simulink model "power_kundur_statcom01"  (R2021a)
settings: Solver=ode23tb  StartTime=0.0  StopTime=10  MaxStep=1/60  RelTol=1e-4  EnableMultiTasking=on
values from neighbouring files (symbols this model uses):
  j = 1    [OABC_PSO_TUNED_NOFault.mat]    (also in OABC_PSO_TUNED_ThreePHASEFault.mat; Traditional_ABC_PSO2.m = randi([1 noFood], 1))
  kk = [0 0.302628193662]    [OABC_PSO_TUNED_NOFault.mat]    (also in OABC_PSO_TUNED_ThreePHASEFault.mat = [6.69502367045 1584.585174])
undefined symbols (not defined in the file or in its folder): Ac, Bc, Cc, D1, Dc, Delta, Fnom, gcbh, K_Vdq2m_SH, Kf_I_SH, Ki_I_SH, Ki_Vac_SH, Ki_Vdc_SH, Kp_I_SH, Kp_Vac_SH, Kp_Vdc_SH, L_RL_SH, MagIinit_SH, PhaIinit_SH, R_RL_SH, sps_rtmsupport, VdcRef_SH, Vnom_SH, xfo_ratio_SH
libraries: spsGenericPowerSystemStabilizerLib x8, spsLoadFlowBusLib x6, spsThreePhaseParallelRLCLoadLib x4, spsThreePhasePISectionLineLib x4, spsSynchronousMachinepuStandardLib x4, spsExcitationSystemLib x4, spsMultiBandPowerSystemStabilizerLib x4, spsSteamTurbineandGovernorLib x4, spsThreePhaseTransformerTwoWindingsLib x4, spsThreePhaseVIMeasurementLib x3, spsThreePhaseBreakerLib x2, spsControlledCurrentSourceLib x2
(part 2 of 3)

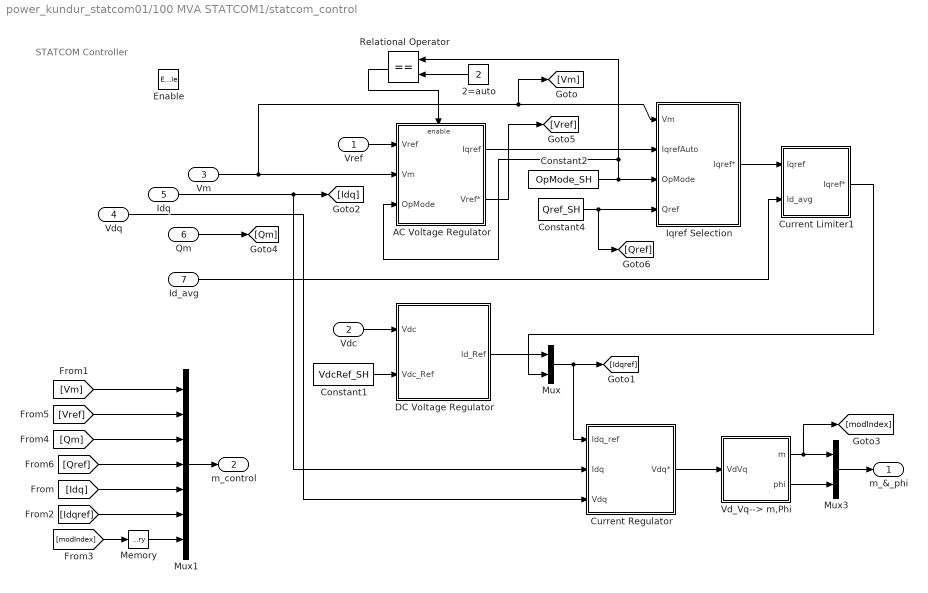
== system power_kundur_statcom01/100 MVA STATCOM1/statcom_control ==
  note: STATCOM Controller
  Vref : Inport
  Vdc : Inport  Port=2  PortDimensions=1
  Vm : Inport  Port=3  PortDimensions=1  SampleTime=0
  Vdq : Inport  Port=4  PortDimensions=2  SampleTime=0
  Idq : Inport  Port=5  PortDimensions=2  SampleTime=0
  Qm : Inport  Port=6  PortDimensions=1  SampleTime=0
  Id_avg : Inport  Port=7  PortDimensions=1  SampleTime=0
  Enable : EnablePort  PropagateVarSize=During execution
  2=auto : Constant  Value=2
  AC Voltage Regulator : Subsystem  mask(PI Controller){Droop=Droop_SH, MaxRateChangeVref_SH=MaxRateChangeVref_SH, Kp=Kp_Vac_SH, Ki=Ki_Vac_SH, Par_Limits=[1 -1], Init=0}
      mask prompts: Droop "Droop (pu):"; MaxRateChangeVref_SH "Maximum rate of change of reference voltage Vref (pu/s):"; Kp "Proportional gain (Kp):"; Ki "Integral gain (Ki):"; Par_Limits "Output limits: [ Upper   Lower ]"; Init "Output initial value:"
      mask help: This block implements a PI controller.
      mask init:
      | UpperLimit=Par_Limits(1);
      | LowerLimit=Par_Limits(2);
  Constant1 : Constant  Value=VdcRef_SH
  Constant2 : Constant  Value=OpMode_SH
  Constant4 : Constant  Value=Qref_SH
  Current Regulator : Subsystem  mask(Current Regulator){Kp_I=Kp_I_SH, Ki_I=Ki_I_SH, Kf_I=Kf_I_SH, ParLimits=[1 -1], Init=0}
      mask prompts: Kp_I "Proportional gain (Kp):"; Ki_I "Integral gain (ki):"; Kf_I "Feedforward decoupling gain (Kf):"; ParLimits "Output limits: [ Upper   Lower ]:"; Init "Output initial value:"
      mask init:
      | UpperLimit=ParLimits(1);
      | LowerLimit=ParLimits(2);
  Current Limiter1 : Subsystem
  DC Voltage Regulator : Subsystem  mask(DC Voltage regulator){Kp=Kp_Vdc_SH, Ki=Ki_Vdc_SH}
      mask prompts: Kp "Proportional gain (Kp):"; Ki "Integral gain(Ki)"
  Iqref Selection : Subsystem
  Memory : Memory  InitialCondition=0.8
  Mux : Mux  Inputs=2
  Mux1 : Mux  Inputs=[1 1 1 1 2 2 1]
  Mux3 : Mux  Inputs=2
  Relational Operator : RelationalOperator  Operator===  RndMeth=Nearest
  Vd_Vq--> m,Phi : Subsystem
  m_&_phi : Outport  InitialOutput=[0]  VectorParamsAs1DForOutWhenUnconnected=off
  m_control : Outport  Port=2  InitialOutput=[0]  VectorParamsAs1DForOutWhenUnconnected=off
  wires:
  Vdc/1 -> DC Voltage Regulator/1(Vdc)
  Constant4/1 -> Iqref Selection/4(Qref), [Qref]
  AC Voltage Regulator/1(Iqref) -> Iqref Selection/2(IqrefAuto)
  Mux1/1 -> m_control/1
  [Vm] -> Mux1/1
  Current Regulator/1(Vdq*) -> Vd_Vq--> m,Phi/1(VdVq)
  Idq/1 -> [Idq], Current Regulator/2(Idq)
  Constant1/1 -> DC Voltage Regulator/2(Vdc_Ref)
  [modIndex] -> Memory/1
  Mux3/1 -> m_&_phi/1
  Vm/1 -> Iqref Selection/1(Vm), [Vm], AC Voltage Regulator/2(Vm)
  Constant2/1 -> Iqref Selection/3(OpMode), AC Voltage Regulator/3(OpMode), Relational Operator/1
  AC Voltage Regulator/2(Vref*) -> [Vref]
  [Vref] -> Mux1/2
  [Qref] -> Mux1/4
  [Qm] -> Mux1/3
  [Idq] -> Mux1/5
  [Idqref] -> Mux1/6
  Memory/1 -> Mux1/7
  Vref/1 -> AC Voltage Regulator/1(Vref)
  DC Voltage Regulator/1(Id_Ref) -> Mux/1
  Mux/1 -> Current Regulator/1(Idq_ref), [Idqref]
  Vdq/1 -> Current Regulator/3(Vdq)
  Vd_Vq--> m,Phi/1(m) -> Mux3/1, [modIndex]
  Vd_Vq--> m,Phi/2(phi) -> Mux3/2
  2=auto/1 -> Relational Operator/2
  Relational Operator/1 -> AC Voltage Regulator/Enable
  Iqref Selection/1(Iqref*) -> Current Limiter1/1(Iqref)
  Current Limiter1/1(Iqref*) -> Mux/2
  Id_avg/1 -> Current Limiter1/2(Id_avg)
  Qm/1 -> [Qm]

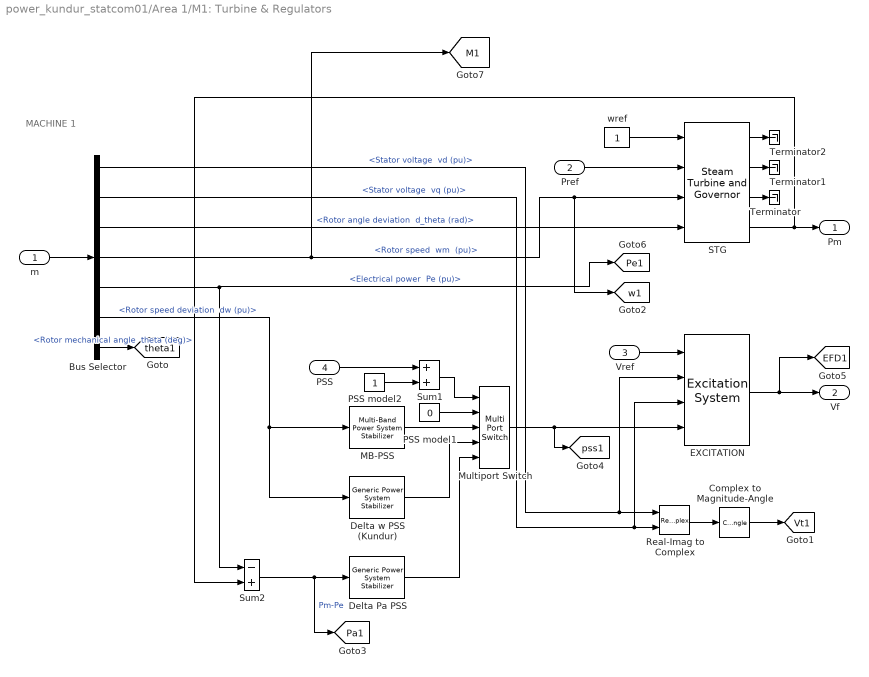
== system power_kundur_statcom01/Area 1/M1: Turbine & Regulators ==
  note: MACHINE 1
  m : Inport
  Pref : Inport  Port=2
  Vref : Inport  Port=3
  PSS : Inport  Port=4
  Bus Selector : BusSelector  OutputSignals="dq0 components.Stator voltage  vd (pu),dq0 components.Stator voltage  vq (pu),Mechanical.Rotor angle deviation  d_theta (rad),Mechanical.Rotor speed  wm  (pu),Mechanical.Electrical power  Pe (pu),Mechanical.Rotor speed deviation  dw (pu),Mechanical.Rotor mechanical angle  theta (deg)"
  Complex to Magnitude-Angle : ComplexToMagnitudeAngle  Output=Magnitude
  "Delta Pa PSS " : spsGenericPowerSystemStabilizerLib/Generic Power System Stabilizer  Tsensor=15e-3  K=2.5*1.25  Twashout=1  Tleadlag1=[60e-3 1]  Tleadlag2=[0 0]  VSlimits=[-0.15 0.15]  Vinit=0  Plot_On=off  MagdB_On=off  FreqRange=logspace(-2,2,500)
      settings: SourceProductBaseCode=PS
  "Delta w PSS (Kundur) " : spsGenericPowerSystemStabilizerLib/Generic Power System Stabilizer  Tsensor=15e-3  K=30  Twashout=10  Tleadlag1=[50e-3 20e-3]  Tleadlag2=[3 5.4]  VSlimits=[-0.15 0.15]  Vinit=0  Plot_On=off  MagdB_On=off  FreqRange=logspace(-2,2,500)
      settings: SourceProductBaseCode=PS
  EXCITATION : spsExcitationSystemLib/Excitation System  tr=20e-3  reg=[ 200, 0.001 ]  exc=[ 1, 0 ]  tgr=[ 0, 0 ]  damp=[ 0, 0 ]  sat=[ 0, 0 ]  lim=[ 0 , 12.3, 0 ]  v0=[1,1.83395]
      settings: SourceProductBaseCode=PS
  "MB-PSS " : spsMultiBandPowerSystemStabilizerLib/Multi-Band Power System Stabilizer  OperationMode=Detailed settings  Kg=1.0  GL=[0.2 30]  GI=[1.25 40]  GH=[12.0 160]  GLd=[66 66 9.4]  TcLF=[1.667 2 0 0 0 0 2 2.4 0 0 0 0 1 1]  GId=[66 66 47.6]  TcIF=[1 1 0.25 0.3 0 0 1 1 0.3 0.36 0 0 0 0]  GHd=[66 66 233]  TcHF="[0.01 0.012 0 0 0 0  0.012 0.0144 0 0 0 0 1 1]"  LIM=[.075 .15 .15 .15]  Plot_On=off  MagdB_On=on  FreqRange=logspace(-2,2,500)
      settings: SourceProductBaseCode=PS
  Multiport Switch : MultiPortSwitch  Inputs=4  InputSameDT=on
  PSS model1 : Constant  Value=0
  PSS model2 : Constant
  Real-Imag to Complex : RealImagToComplex
  STG : spsSteamTurbineandGovernorLib/Steam Turbine and Governor  gentype=Tandem-compound (single mass)  reg1="[ 1  0.05    0 ]"  reg2="[ 0.001  0.15 ]"  reg3="[ -0.1  0.1  0  4.496 ]"  N=3600  turb1="[ 0  10   3.3   0.5   ]"  turb2="[   0   0.36    0.36   0.28   ]"  HA="[ 0.046  1.430  1.465   0.192 ]"  KA="[ 90.44  53.88  64.59   62.94  ]"  DA="[ 0.0115  0.3575  0.3663   0.0137  ]"  ini1=0.7778  ini2=[0.779316,-31.4247]
      settings: SourceProductBaseCode=PS
  Sum1 : Sum  InputSameDT=on  SaturateOnIntegerOverflow=on  OutDataTypeStr=Inherit: Same as first input
  Sum2 : Sum  Inputs=-+  InputSameDT=on  SaturateOnIntegerOverflow=on  OutDataTypeStr=Inherit: Same as first input
  Terminator : Terminator
  Terminator1 : Terminator
  Terminator2 : Terminator
  wref : Constant
  Pm : Outport  InitialOutput=0
  Vf : Outport  Port=2  InitialOutput=0
  tag scope: EFD1=global, M1=global, Pa1=global, Pe1=global, Vt1=global, pss1=global, theta1=global, w1=global
  wires:
  Bus Selector/1 -> Real-Imag to Complex/1, EXCITATION/2  "<Stator voltage  vd (pu)>"
  Bus Selector/2 -> Real-Imag to Complex/2, EXCITATION/3  "<Stator voltage  vq (pu)>"
  wref/1 -> STG/1
  Pref/1 -> STG/2
  m/1 -> Bus Selector/1
  Vref/1 -> EXCITATION/1
  Real-Imag to Complex/1 -> Complex to Magnitude-Angle/1
  EXCITATION/1 -> Vf/1, [EFD1]
  Complex to Magnitude-Angle/1 -> [Vt1]
  Bus Selector/7 -> [theta1]  "<Rotor mechanical angle  theta (deg)>"
  Multiport Switch/1 -> EXCITATION/4, [pss1]
  PSS model1/1 -> Multiport Switch/2
  "MB-PSS "/1 -> Multiport Switch/3
  "Delta w PSS (Kundur) "/1 -> Multiport Switch/4
  "Delta Pa PSS "/1 -> Multiport Switch/5
  PSS model2/1 -> Sum1/2
  Sum1/1 -> Multiport Switch/1
  PSS/1 -> Sum1/1
  Bus Selector/4 -> [M1], [w1], STG/3  "<Rotor speed  wm  (pu)>"
  Bus Selector/5 -> [Pe1], Sum2/1  "<Electrical power  Pe (pu)>"
  Bus Selector/6 -> "Delta w PSS (Kundur) "/1, "MB-PSS "/1  "<Rotor speed deviation  dw (pu)>"
  Sum2/1 -> [Pa1], "Delta Pa PSS "/1  "Pm-Pe"
  STG/3 -> Terminator/1
  STG/4 -> Pm/1, Sum2/2
  STG/2 -> Terminator1/1
  STG/1 -> Terminator2/1
  Bus Selector/3 -> STG/4  "<Rotor angle deviation  d_theta (rad)>"

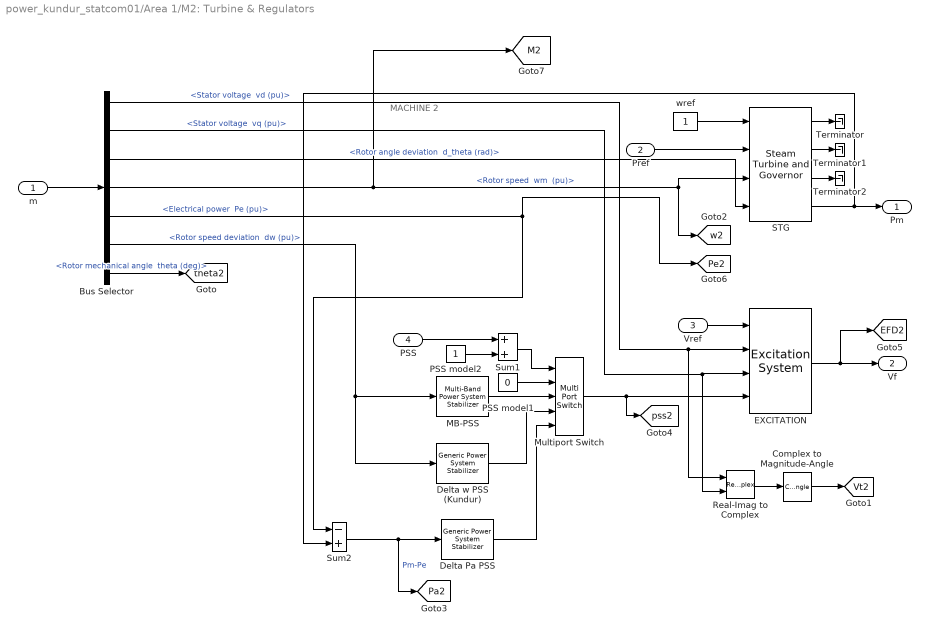
== system power_kundur_statcom01/Area 1/M2: Turbine & Regulators ==
  note: MACHINE 2
  m : Inport
  Pref : Inport  Port=2
  Vref : Inport  Port=3
  PSS : Inport  Port=4
  Bus Selector : BusSelector  OutputSignals="dq0 components.Stator voltage  vd (pu),dq0 components.Stator voltage  vq (pu),Mechanical.Rotor angle deviation  d_theta (rad),Mechanical.Rotor speed  wm  (pu),Mechanical.Electrical power  Pe (pu),Mechanical.Rotor speed deviation  dw (pu),Mechanical.Rotor mechanical angle  theta (deg)"
  Complex to Magnitude-Angle : ComplexToMagnitudeAngle  Output=Magnitude
  "Delta Pa PSS " : spsGenericPowerSystemStabilizerLib/Generic Power System Stabilizer  Tsensor=15e-3  K=2.5*1.25  Twashout=1  Tleadlag1=[60e-3 1]  Tleadlag2=[0 0]  VSlimits=[-0.15 0.15]  Vinit=0  Plot_On=off  MagdB_On=on  FreqRange=logspace(-2,2,500)
      settings: SourceProductBaseCode=PS
  "Delta w PSS (Kundur) " : spsGenericPowerSystemStabilizerLib/Generic Power System Stabilizer  Tsensor=15e-3  K=30  Twashout=10  Tleadlag1=[50e-3 20e-3]  Tleadlag2=[3 5.4]  VSlimits=[-0.15 0.15]  Vinit=0  Plot_On=off  MagdB_On=on  FreqRange=logspace(-2,2,500)
      settings: SourceProductBaseCode=PS
  EXCITATION : spsExcitationSystemLib/Excitation System  tr=20e-3  reg=[ 200, 0.001 ]  exc=[ 1, 0 ]  tgr=[ 0, 0 ]  damp=[ 0, 0 ]  sat=[ 0, 0 ]  lim=[ 0 , 12.3, 0 ]  v0=[1,1.86756]
      settings: SourceProductBaseCode=PS
  "MB-PSS " : spsMultiBandPowerSystemStabilizerLib/Multi-Band Power System Stabilizer  OperationMode=Simplified settings  Kg=1.0  GL=[0.2 30]  GI=[1.25 40]  GH=[12.0 160]  GLd=[66 66 9.4]  TcLF=[1.667 2 0 0 0 0 2 2.4 0 0 0 0 1 1]  GId=[66 66 47.6]  TcIF=[1 1 0.25 0.3 0 0 1 1 0.3 0.36 0 0 0 0]  GHd=[66 66 233]  TcHF="[0.01 0.012 0 0 0 0  0.012 0.0144 0 0 0 0 1 1]"  LIM=[.075 .15 .15 .15]  Plot_On=off  MagdB_On=off  FreqRange=logspace(-2,2,500)
      settings: SourceProductBaseCode=PS
  Multiport Switch : MultiPortSwitch  Inputs=4  InputSameDT=on
  PSS model1 : Constant  Value=0
  PSS model2 : Constant
  Real-Imag to Complex : RealImagToComplex
  STG : spsSteamTurbineandGovernorLib/Steam Turbine and Governor  gentype=Tandem-compound (single mass)  reg1="[ 1  0.05    0 ]"  reg2="[ 0.001  0.15 ]"  reg3="[ -0.1  0.1  0  4.496 ]"  N=3600  turb1="[ 0  10   3.3   0.5   ]"  turb2="[   0   0.36    0.36   0.28   ]"  HA="[ 0.046  1.430  1.465   0.192 ]"  KA="[ 90.44  53.88  64.59   62.94  ]"  DA="[ 0.0115  0.3575  0.3663   0.0137  ]"  ini1=0.7777  ini2=[0.779243,-42.8075]
      settings: SourceProductBaseCode=PS
  Sum1 : Sum  InputSameDT=on  SaturateOnIntegerOverflow=on  OutDataTypeStr=Inherit: Same as first input
  Sum2 : Sum  Inputs=-+  InputSameDT=on  SaturateOnIntegerOverflow=on  OutDataTypeStr=Inherit: Same as first input
  Terminator : Terminator
  Terminator1 : Terminator
  Terminator2 : Terminator
  wref : Constant
  Pm : Outport  InitialOutput=0
  Vf : Outport  Port=2  InitialOutput=0
  tag scope: EFD2=global, M2=global, Pa2=global, Pe2=global, Vt2=global, pss2=global, theta2=global, w2=global
  wires:
  Sum2/1 -> [Pa2], "Delta Pa PSS "/1  "Pm-Pe"
  Bus Selector/6 -> "MB-PSS "/1, "Delta w PSS (Kundur) "/1  "<Rotor speed deviation  dw (pu)>"
  Bus Selector/5 -> [Pe2], Sum2/1  "<Electrical power  Pe (pu)>"
  Bus Selector/4 -> [M2], STG/3, [w2]  "<Rotor speed  wm  (pu)>"
  PSS/1 -> Sum1/1
  Sum1/1 -> Multiport Switch/1
  PSS model2/1 -> Sum1/2
  "Delta Pa PSS "/1 -> Multiport Switch/5
  "Delta w PSS (Kundur) "/1 -> Multiport Switch/4
  "MB-PSS "/1 -> Multiport Switch/3
  PSS model1/1 -> Multiport Switch/2
  Multiport Switch/1 -> [pss2], EXCITATION/4
  Bus Selector/7 -> [theta2]  "<Rotor mechanical angle  theta (deg)>"
  Complex to Magnitude-Angle/1 -> [Vt2]
  EXCITATION/1 -> [EFD2], Vf/1
  Real-Imag to Complex/1 -> Complex to Magnitude-Angle/1
  Vref/1 -> EXCITATION/1
  Pref/1 -> STG/2
  wref/1 -> STG/1
  Bus Selector/2 -> Real-Imag to Complex/2, EXCITATION/3  "<Stator voltage  vq (pu)>"
  Bus Selector/1 -> Real-Imag to Complex/1, EXCITATION/2  "<Stator voltage  vd (pu)>"
  STG/1 -> Terminator/1
  STG/2 -> Terminator1/1
  STG/3 -> Terminator2/1
  STG/4 -> Pm/1, Sum2/2
  Bus Selector/3 -> STG/4  "<Rotor angle deviation  d_theta (rad)>"
  m/1 -> Bus Selector/1

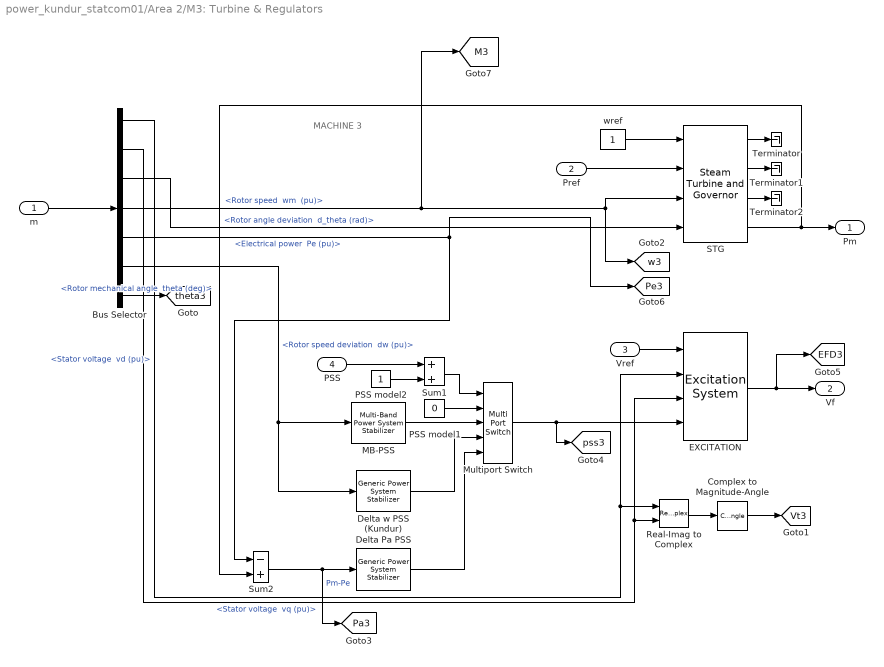
== system power_kundur_statcom01/Area 2/M3: Turbine & Regulators ==
  note: MACHINE 3
  m : Inport
  Pref : Inport  Port=2
  Vref : Inport  Port=3
  PSS : Inport  Port=4
  Bus Selector : BusSelector  OutputSignals="dq0 components.Stator voltage  vd (pu),dq0 components.Stator voltage  vq (pu),Mechanical.Rotor angle deviation  d_theta (rad),Mechanical.Rotor speed  wm  (pu),Mechanical.Electrical power  Pe (pu),Mechanical.Rotor speed deviation  dw (pu),Mechanical.Rotor mechanical angle  theta (deg)"
  Complex to Magnitude-Angle : ComplexToMagnitudeAngle  Output=Magnitude
  "Delta Pa PSS " : spsGenericPowerSystemStabilizerLib/Generic Power System Stabilizer  Tsensor=15e-3  K=2.5*1.25  Twashout=1  Tleadlag1=[60e-3 1]  Tleadlag2=[0 0]  VSlimits=[-0.15 0.15]  Vinit=0  Plot_On=off  MagdB_On=on  FreqRange=logspace(-2,2,500)
      settings: SourceProductBaseCode=PS
  "Delta w PSS (Kundur) " : spsGenericPowerSystemStabilizerLib/Generic Power System Stabilizer  Tsensor=15e-3  K=30  Twashout=10  Tleadlag1=[50e-3 20e-3]  Tleadlag2=[3 5.4]  VSlimits=[-0.15 0.15]  Vinit=0  Plot_On=off  MagdB_On=on  FreqRange=logspace(-2,2,500)
      settings: SourceProductBaseCode=PS
  EXCITATION : spsExcitationSystemLib/Excitation System  tr=20e-3  reg=[ 200, 0.001 ]  exc=[ 1, 0 ]  tgr=[ 0, 0 ]  damp=[ 0, 0 ]  sat=[ 0, 0 ]  lim=[ 0 , 12.3, 0 ]  v0=[1,1.85092]
      settings: SourceProductBaseCode=PS
  "MB-PSS " : spsMultiBandPowerSystemStabilizerLib/Multi-Band Power System Stabilizer  OperationMode=Simplified settings  Kg=1.0  GL=[0.2 30]  GI=[1.25 40]  GH=[12.0 160]  GLd=[66 66 9.4]  TcLF=[1.667 2 0 0 0 0 2 2.4 0 0 0 0 1 1]  GId=[66 66 47.6]  TcIF=[1 1 0.25 0.3 0 0 1 1 0.3 0.36 0 0 0 0]  GHd=[66 66 233]  TcHF="[0.01 0.012 0 0 0 0  0.012 0.0144 0 0 0 0 1 1]"  LIM=[.075 .15 .15 .15]  Plot_On=off  MagdB_On=off  FreqRange=logspace(-2,2,500)
      settings: SourceProductBaseCode=PS
  Multiport Switch : MultiPortSwitch  Inputs=4  InputSameDT=on
  PSS model1 : Constant  Value=0
  PSS model2 : Constant
  Real-Imag to Complex : RealImagToComplex
  STG : spsSteamTurbineandGovernorLib/Steam Turbine and Governor  gentype=Tandem-compound (single mass)  reg1="[ 1  0.05    0 ]"  reg2="[ 0.001  0.15 ]"  reg3="[ -0.1  0.1  0  4.496 ]"  N=3600  turb1="[ 0  10   3.3   0.5   ]"  turb2="[   0   0.36    0.36   0.28   ]"  HA="[ 0.046  1.430  1.465   0.192 ]"  KA="[ 90.44  53.88  64.59   62.94  ]"  DA="[ 0.0115  0.3575  0.3663   0.0137  ]"  ini1=0.798889  ini2=[0.800505,-56.3243]
      settings: SourceProductBaseCode=PS
  Sum1 : Sum  InputSameDT=on  SaturateOnIntegerOverflow=on  OutDataTypeStr=Inherit: Same as first input
  Sum2 : Sum  Inputs=-+  InputSameDT=on  SaturateOnIntegerOverflow=on  OutDataTypeStr=Inherit: Same as first input
  Terminator : Terminator
  Terminator1 : Terminator
  Terminator2 : Terminator
  wref : Constant
  Pm : Outport  InitialOutput=0
  Vf : Outport  Port=2  InitialOutput=0
  tag scope: EFD3=global, M3=global, Pa3=global, Pe3=global, Vt3=global, pss3=global, theta3=global, w3=global
  wires:
  Sum2/1 -> [Pa3], "Delta Pa PSS "/1  "Pm-Pe"
  Bus Selector/6 -> "MB-PSS "/1, "Delta w PSS (Kundur) "/1  "<Rotor speed deviation  dw (pu)>"
  Bus Selector/5 -> [Pe3], Sum2/1  "<Electrical power  Pe (pu)>"
  Bus Selector/4 -> [M3], STG/3, [w3]  "<Rotor speed  wm  (pu)>"
  PSS/1 -> Sum1/1
  Sum1/1 -> Multiport Switch/1
  PSS model2/1 -> Sum1/2
  "Delta Pa PSS "/1 -> Multiport Switch/5
  "Delta w PSS (Kundur) "/1 -> Multiport Switch/4
  "MB-PSS "/1 -> Multiport Switch/3
  PSS model1/1 -> Multiport Switch/2
  Multiport Switch/1 -> [pss3], EXCITATION/4
  Bus Selector/7 -> [theta3]  "<Rotor mechanical angle  theta (deg)>"
  Complex to Magnitude-Angle/1 -> [Vt3]
  EXCITATION/1 -> [EFD3], Vf/1
  Real-Imag to Complex/1 -> Complex to Magnitude-Angle/1
  Vref/1 -> EXCITATION/1
  Pref/1 -> STG/2
  wref/1 -> STG/1
  Bus Selector/2 -> EXCITATION/3, Real-Imag to Complex/2  "<Stator voltage  vq (pu)>"
  Bus Selector/1 -> EXCITATION/2, Real-Imag to Complex/1  "<Stator voltage  vd (pu)>"
  Bus Selector/3 -> STG/4  "<Rotor angle deviation  d_theta (rad)>"
  STG/1 -> Terminator/1
  STG/2 -> Terminator1/1
  STG/3 -> Terminator2/1
  STG/4 -> Pm/1, Sum2/2
  m/1 -> Bus Selector/1

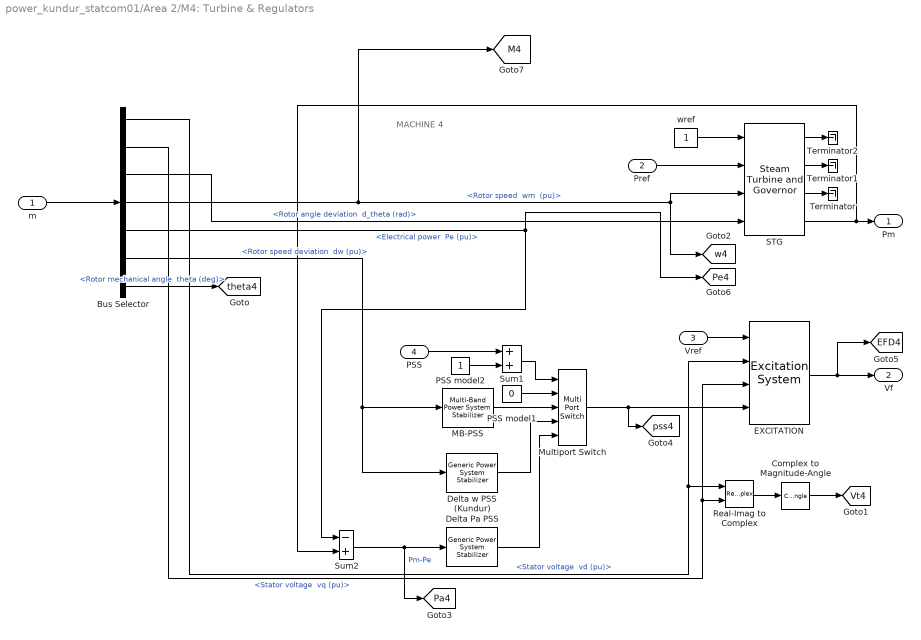
== system power_kundur_statcom01/Area 2/M4: Turbine & Regulators ==
  note: MACHINE 4
  m : Inport
  Pref : Inport  Port=2
  Vref : Inport  Port=3
  PSS : Inport  Port=4
  Bus Selector : BusSelector  OutputSignals="dq0 components.Stator voltage  vd (pu),dq0 components.Stator voltage  vq (pu),Mechanical.Rotor angle deviation  d_theta (rad),Mechanical.Rotor speed  wm  (pu),Mechanical.Electrical power  Pe (pu),Mechanical.Rotor speed deviation  dw (pu),Mechanical.Rotor mechanical angle  theta (deg)"
  Complex to Magnitude-Angle : ComplexToMagnitudeAngle  Output=Magnitude
  "Delta Pa PSS " : spsGenericPowerSystemStabilizerLib/Generic Power System Stabilizer  Tsensor=15e-3  K=2.5*1.25  Twashout=1  Tleadlag1=[60e-3 1]  Tleadlag2=[0 0]  VSlimits=[-0.15 0.15]  Vinit=0  Plot_On=off  MagdB_On=on  FreqRange=logspace(-2,2,500)
      settings: SourceProductBaseCode=PS
  "Delta w PSS (Kundur) " : spsGenericPowerSystemStabilizerLib/Generic Power System Stabilizer  Tsensor=15e-3  K=30  Twashout=10  Tleadlag1=[50e-3 20e-3]  Tleadlag2=[3 5.4]  VSlimits=[-0.15 0.15]  Vinit=0  Plot_On=off  MagdB_On=on  FreqRange=logspace(-2,2,500)
      settings: SourceProductBaseCode=PS
  EXCITATION : spsExcitationSystemLib/Excitation System  tr=20e-3  reg=[ 200, 0.001 ]  exc=[ 1, 0 ]  tgr=[ 0, 0 ]  damp=[ 0, 0 ]  sat=[ 0, 0 ]  lim=[ 0 , 12.3, 0 ]  v0=[1,1.82209]
      settings: SourceProductBaseCode=PS
  "MB-PSS " : spsMultiBandPowerSystemStabilizerLib/Multi-Band Power System Stabilizer  OperationMode=Simplified settings  Kg=1.0  GL=[0.2 30]  GI=[1.25 40]  GH=[12.0 160]  GLd=[66 66 9.4]  TcLF=[1.667 2 0 0 0 0 2 2.4 0 0 0 0 1 1]  GId=[66 66 47.6]  TcIF=[1 1 0.25 0.3 0 0 1 1 0.3 0.36 0 0 0 0]  GHd=[66 66 233]  TcHF="[0.01 0.012 0 0 0 0  0.012 0.0144 0 0 0 0 1 1]"  LIM=[.075 .15 .15 .15]  Plot_On=off  MagdB_On=off  FreqRange=logspace(-2,2,500)
      settings: SourceProductBaseCode=PS
  Multiport Switch : MultiPortSwitch  Inputs=4  InputSameDT=on
  PSS model1 : Constant  Value=0
  PSS model2 : Constant
  Real-Imag to Complex : RealImagToComplex
  STG : spsSteamTurbineandGovernorLib/Steam Turbine and Governor  gentype=Tandem-compound (single mass)  reg1="[ 1  0.05    0 ]"  reg2="[ 0.001  0.15 ]"  reg3="[ -0.1  0.1  0  4.496 ]"  N=3600  turb1="[ 0  10   3.3   0.5   ]"  turb2="[   0   0.36    0.36   0.28   ]"  HA="[ 0.046  1.430  1.465   0.192 ]"  KA="[ 90.44  53.88  64.59   62.94  ]"  DA="[ 0.0115  0.3575  0.3663   0.0137  ]"  ini1=0.7778  ini2=[0.779311,-67.7513]
      settings: SourceProductBaseCode=PS
  Sum1 : Sum  InputSameDT=on  SaturateOnIntegerOverflow=on  OutDataTypeStr=Inherit: Same as first input
  Sum2 : Sum  Inputs=-+  InputSameDT=on  SaturateOnIntegerOverflow=on  OutDataTypeStr=Inherit: Same as first input
  Terminator : Terminator
  Terminator1 : Terminator
  Terminator2 : Terminator
  wref : Constant
  Pm : Outport  InitialOutput=0
  Vf : Outport  Port=2  InitialOutput=0
  tag scope: EFD4=global, M4=global, Pa4=global, Pe4=global, Vt4=global, pss4=global, theta4=global, w4=global
  wires:
  Bus Selector/1 -> EXCITATION/2, Real-Imag to Complex/1  "<Stator voltage  vd (pu)>"
  Bus Selector/2 -> EXCITATION/3, Real-Imag to Complex/2  "<Stator voltage  vq (pu)>"
  STG/4 -> Pm/1, Sum2/2
  wref/1 -> STG/1
  Pref/1 -> STG/2
  Vref/1 -> EXCITATION/1
  STG/3 -> Terminator/1
  Real-Imag to Complex/1 -> Complex to Magnitude-Angle/1
  EXCITATION/1 -> Vf/1, [EFD4]
  Complex to Magnitude-Angle/1 -> [Vt4]
  Bus Selector/7 -> [theta4]  "<Rotor mechanical angle  theta (deg)>"
  Multiport Switch/1 -> EXCITATION/4, [pss4]
  PSS model1/1 -> Multiport Switch/2
  "MB-PSS "/1 -> Multiport Switch/3
  "Delta w PSS (Kundur) "/1 -> Multiport Switch/4
  "Delta Pa PSS "/1 -> Multiport Switch/5
  PSS model2/1 -> Sum1/2
  Sum1/1 -> Multiport Switch/1
  PSS/1 -> Sum1/1
  Bus Selector/4 -> [M4], STG/3, [w4]  "<Rotor speed  wm  (pu)>"
  Bus Selector/5 -> [Pe4], Sum2/1  "<Electrical power  Pe (pu)>"
  Bus Selector/6 -> "MB-PSS "/1, "Delta w PSS (Kundur) "/1  "<Rotor speed deviation  dw (pu)>"
  Sum2/1 -> [Pa4], "Delta Pa PSS "/1  "Pm-Pe"
  STG/2 -> Terminator1/1
  STG/1 -> Terminator2/1
  Bus Selector/3 -> STG/4  "<Rotor angle deviation  d_theta (rad)>"
  m/1 -> Bus Selector/1

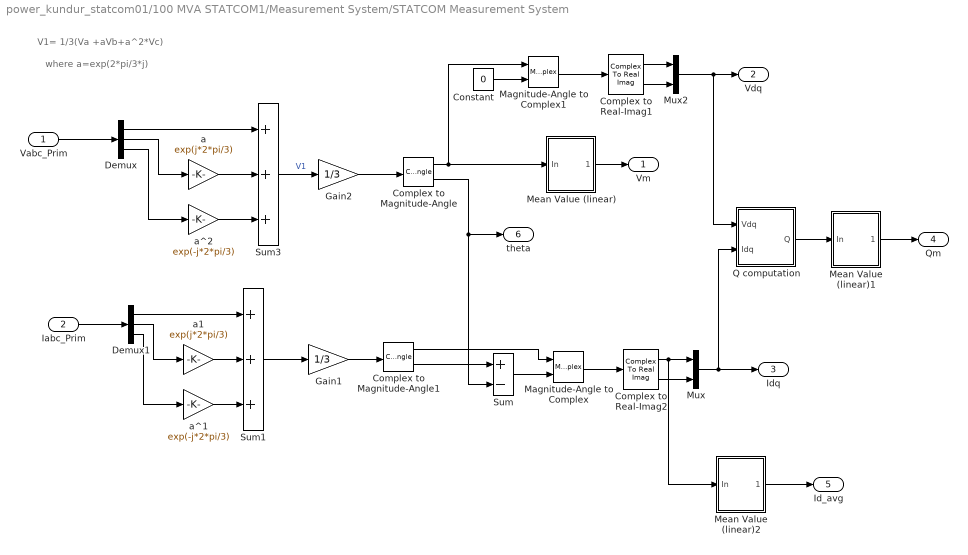
== system power_kundur_statcom01/100 MVA STATCOM1/Measurement System/STATCOM Measurement System ==
  note: where a=exp(2*pi/3*j)
  note: V1= 1/3(Va +aVb+a^2*Vc)
  Vabc_Prim : Inport
  Iabc_Prim : Inport  Port=2
  Complex to Magnitude-Angle : ComplexToMagnitudeAngle
  Complex to Magnitude-Angle1 : ComplexToMagnitudeAngle
  Complex to Real-Imag1 : ComplexToRealImag
  Complex to Real-Imag2 : ComplexToRealImag
  Constant : Constant  Value=0
  Demux : Demux  Outputs=3
      settings: DisplayOption=none
  Demux1 : Demux  Outputs=3
      settings: DisplayOption=none
  Gain1 : Gain  Gain=1/3  SaturateOnIntegerOverflow=on  OutDataTypeStr=Inherit: Same as input  ParamDataTypeStr=Inherit: Same as input
  Gain2 : Gain  Gain=1/3  SaturateOnIntegerOverflow=on  OutDataTypeStr=Inherit: Same as input  ParamDataTypeStr=Inherit: Same as input
  Magnitude-Angle to Complex : MagnitudeAngleToComplex
  Magnitude-Angle to Complex1 : MagnitudeAngleToComplex
  Mean Value (linear) : Subsystem  DialogController=POWERSYS.PowerSysDialog  mask(Mean Value (linear)){Freq=Fnom, n=3, Vinit=Vm_SH_Init}
      mask prompts: Freq "Fundamental frequency (Hz)"; n "Pade order (for linearization)"; Vinit "Initial input:"
      mask help: This block implements a linear model of a measurement system that computes the mean value of the input signal over a running window of one cycle of the specified fundamental frequency. Pade approximation is used to linearize the one-cycle delay introduced by such a running average measurement system . A low order Pade approximation of order 3 is usually sufficient to represent the system dynamic response. However, a high order Pade approximation may be required to achieve an acceptable filtering of harmonics of the input signal.
      mask init:
      | % Pade Approximation:
      | % The coefficients of the Pade approximation are given by the 
      | % recursion   h[k+1] = (N-k)/(2*N-k)/(k+1) * h[k],  h[0] = 1
      | % and 
      | %     exp(-T*s) == Sum { h[k] (-T*s)^k } / Sum { h[k] (T*s)^k }
      | %
      | T=1/Freq;
      | a = zeros(1,n+1);   a(1) = 1;
      | b = zeros(1,n+1);   b(1) = 1;
      | for k = 1:n,
      | 	fact = T*(n-k+1)/(2*n-k+1)/k;
      | 	a(k+1) = (-fact) * a(k);
      | 	b(k+1) = fact * b(k);
      | end
      | a = fliplr(a/b(n+1));
      | b = fliplr(b/b(n+1));
      | %
      | %Initial conditions:
      | [Ac,Bc,Cc,Dc]=tf2ss(a,b);
      | u=Vinit*exp(j*90*pi/180);
      | u0=imag(u); % input at  t=0;
      | I=eye(size(Ac));
      | x=inv(-Ac)*Bc*u;
      | x0c=imag(x);
      | power_initmask();
      mask Help: This block is part of a subset of blocks in the Extras library that does not have documentation associated with it, other than the block mask description.
      mask Display: disp('Mean\n(linear)')
  Mean Value (linear)1 : Subsystem  DialogController=POWERSYS.PowerSysDialog  mask(Mean Value (linear)){Freq=Fnom, n=3, Vinit=Qm_SH_Init}
      mask prompts: Freq "Fundamental frequency (Hz)"; n "Pade order (for linearization)"; Vinit "Initial input:"
      mask help: This block implements a linear model of a measurement system that computes the mean value of the input signal over a running window of one cycle of the specified fundamental frequency. Pade approximation is used to linearize the one-cycle delay introduced by such a running average measurement system . A low order Pade approximation of order 3 is usually sufficient to represent the system dynamic response. However, a high order Pade approximation may be required to achieve an acceptable filtering of harmonics of the input signal.
      mask init: same as power_kundur_statcom01/100 MVA STATCOM1/Measurement System/STATCOM Measurement System/Mean Value (linear)
      mask Help: This block is part of a subset of blocks in the Extras library that does not have documentation associated with it, other than the block mask description.
      mask Display: disp('Mean\n(linear)')
  Mean Value (linear)2 : Subsystem  DialogController=POWERSYS.PowerSysDialog  mask(Mean Value (linear)){Freq=Fnom, n=3, Vinit=Id_avg_SH_Init}
      mask prompts: Freq "Fundamental frequency (Hz)"; n "Pade order (for linearization)"; Vinit "Initial input:"
      mask help: This block implements a linear model of a measurement system that computes the mean value of the input signal over a running window of one cycle of the specified fundamental frequency. Pade approximation is used to linearize the one-cycle delay introduced by such a running average measurement system . A low order Pade approximation of order 3 is usually sufficient to represent the system dynamic response. However, a high order Pade approximation may be required to achieve an acceptable filtering of harmonics of the input signal.
      mask init: same as power_kundur_statcom01/100 MVA STATCOM1/Measurement System/STATCOM Measurement System/Mean Value (linear)
      mask Help: This block is part of a subset of blocks in the Extras library that does not have documentation associated with it, other than the block mask description.
      mask Display: disp('Mean\n(linear)')
  Mux : Mux  Inputs=2
  Mux2 : Mux  Inputs=2
  Q computation : Subsystem
  Sum : Sum  Inputs=+-  SaturateOnIntegerOverflow=on
  Sum1 : Sum  Inputs=+++  InputSameDT=on  SaturateOnIntegerOverflow=on  OutDataTypeStr=Inherit: Same as first input
  Sum3 : Sum  Inputs=+++  InputSameDT=on  SaturateOnIntegerOverflow=on  OutDataTypeStr=Inherit: Same as first input
  a : Gain  Gain=exp(j*2*pi/3)  SaturateOnIntegerOverflow=on  OutDataTypeStr=Inherit: Same as input  ParamDataTypeStr=Inherit: Same as input
  a1 : Gain  Gain=exp(j*2*pi/3)  SaturateOnIntegerOverflow=on  OutDataTypeStr=Inherit: Same as input  ParamDataTypeStr=Inherit: Same as input
  a^1 : Gain  Gain=exp(-j*2*pi/3)  SaturateOnIntegerOverflow=on  OutDataTypeStr=Inherit: Same as input  ParamDataTypeStr=Inherit: Same as input
  a^2 : Gain  Gain=exp(-j*2*pi/3)  SaturateOnIntegerOverflow=on  OutDataTypeStr=Inherit: Same as input  ParamDataTypeStr=Inherit: Same as input
  Vm : Outport  VectorParamsAs1DForOutWhenUnconnected=off
  Vdq : Outport  Port=2  VectorParamsAs1DForOutWhenUnconnected=off
  Idq : Outport  Port=3  VectorParamsAs1DForOutWhenUnconnected=off
  Qm : Outport  Port=4  VectorParamsAs1DForOutWhenUnconnected=off
  Id_avg : Outport  Port=5  VectorParamsAs1DForOutWhenUnconnected=off
  theta : Outport  Port=6  VectorParamsAs1DForOutWhenUnconnected=off
  wires:
  Constant/1 -> Magnitude-Angle to Complex1/2
  Mux2/1 -> Q computation/1(Vdq), Vdq/1
  Magnitude-Angle to Complex1/1 -> Complex to Real-Imag1/1
  Complex to Real-Imag1/2 -> Mux2/2
  Complex to Real-Imag1/1 -> Mux2/1
  Mux/1 -> Q computation/2(Idq), Idq/1
  Complex to Real-Imag2/2 -> Mux/2
  Complex to Real-Imag2/1 -> Mux/1, Mean Value (linear)2/1(In)
  Magnitude-Angle to Complex/1 -> Complex to Real-Imag2/1
  Complex to Magnitude-Angle1/1 -> Magnitude-Angle to Complex/1
  Sum/1 -> Magnitude-Angle to Complex/2
  Complex to Magnitude-Angle1/2 -> Sum/1
  Gain1/1 -> Complex to Magnitude-Angle1/1
  Complex to Magnitude-Angle/1 -> Magnitude-Angle to Complex1/1, Mean Value (linear)/1(In)
  Iabc_Prim/1 -> Demux1/1
  Sum1/1 -> Gain1/1
  Demux1/1 -> Sum1/1
  a1/1 -> Sum1/2
  a^1/1 -> Sum1/3
  Demux1/2 -> a1/1
  Demux1/3 -> a^1/1
  Gain2/1 -> Complex to Magnitude-Angle/1
  Demux/3 -> a^2/1
  Demux/2 -> a/1
  a^2/1 -> Sum3/3
  a/1 -> Sum3/2
  Demux/1 -> Sum3/1
  Sum3/1 -> Gain2/1  "V1"
  Vabc_Prim/1 -> Demux/1
  Complex to Magnitude-Angle/2 -> theta/1, Sum/2
  Mean Value (linear)/1(Mean) -> Vm/1
  Q computation/1(Q) -> Mean Value (linear)1/1(In)
  Mean Value (linear)1/1(Mean) -> Qm/1
  Mean Value (linear)2/1(Mean) -> Id_avg/1

== system power_kundur_statcom01/100 MVA STATCOM1/Power Components Modeling (Shunt & Series Converter)/Power Components modeling (Shunt Converter) ==
  Vabc_Conv : Inport  PortDimensions=3
  Vabc_prim : Inport  Port=2  PortDimensions=3
  Trip_SH : Inport  Port=3  PortDimensions=1
  Constant1 : Constant  Value=1e6
  Constant2 : Constant  Value=R_RL_SH
  Demux1 : Demux  Outputs=2
      settings: DisplayOption=none
  Ia : spsControlledCurrentSourceLib/Controlled Current Source  Description=source block  Initialize=on  Source_Type=AC  Amplitude=MagIinit_SH  Phase=PhaIinit_SH  Frequency=Fnom  Measurements=None
  Ib : spsControlledCurrentSourceLib/Controlled Current Source  Description=source block  Initialize=on  Source_Type=AC  Amplitude=MagIinit_SH  Phase=PhaIinit_SH-120  Frequency=Fnom  Measurements=None
  Switch3 : Switch  Threshold=0.5  SaturateOnIntegerOverflow=on
  dq-axis model of 3-ph RL branch : Subsystem  mask{Fnom=Fnom, Pnom=Pnom_SH, Vnom=Vnom_SH, R_RL=R_RL_SH, L_RL=L_RL_SH}
      mask prompts: Fnom "Nominal frequency (HZ):"; Pnom "Nominal power (VA):"; Vnom "Nominal voltage (Vrms L-L)"; R_RL "Resistance (pu)"; L_RL "Inductance (pu)"
  A : PMIOPort  Side=Left
  B : PMIOPort  Port=2  Side=Left
  C : PMIOPort  Port=3  Side=Left
  wires:
  Demux1/1 -> Ia/1
  Demux1/2 -> Ib/1
  dq-axis model of 3-ph RL branch/1(Ia_Ib) -> Demux1/1
  Vabc_prim/1 -> dq-axis model of 3-ph RL branch/1(V1abc)
  Vabc_Conv/1 -> dq-axis model of 3-ph RL branch/2(V2abc)
  Switch3/1 -> dq-axis model of 3-ph RL branch/3(R_RL)
  Trip_SH/1 -> Switch3/2
  Constant2/1 -> Switch3/3
  Constant1/1 -> Switch3/1
  connections:
  C/RConn1 -- Ia/RConn1 -- Ib/RConn1
  A/RConn1 -- Ia/LConn1
  B/RConn1 -- Ib/LConn1

== system power_kundur_statcom01/100 MVA STATCOM1/statcom_control/AC Voltage Regulator ==
  note: 2=Auto
  Vref : Inport
  Vm : Inport  Port=2
  OpMode : Inport  Port=3
  Enable : EnablePort  PropagateVarSize=During execution
  1st-Order Filter : Subsystem  DialogController=POWERSYS.PowerSysDialog  mask(First-Order Filter){FilterType=Lowpass, Tc=100e-6, Initialize=off, Vac_Init=[0.8 -25 60], Vdc_Init=-0.4, PlotResponse=off, param1=[1 500 1]}
      mask prompts: FilterType "Filter Type:"; Tc "Time constant (s):"; Initialize "Initialize filter states"; Vac_Init "AC initial input: [ Mag  Phase(degrees)  Freq(Hz) ]"; Vdc_Init "DC Initial input:"; PlotResponse "Plot filter response"; param1 "Frequency range(Hz) : [Start  End  Inc.]"
      mask init:
      | switch FilterType
      | case 1, % Lowpass
      |        X=[0 1 2 3 4];
      |        Y=[-2 -2 -3 -4 -4];
      |        numc=1;
      |        denc=[Tc 1];
      |  case 2,   % Highpass
      |        X=[0 1 2 3 4];
      |        Y=[-4 -4 -3 -2 -2];
      |         numc=[1 0];
      |         denc=[1 1/Tc];
      | end
      | %
      | [Ac,Bc,Cc,Dc]=tf2ss(numc,denc);
      | %
      | %
      | if Initialize==1  % Compute initial conditions on states
      | u1=Vac_Init(1)*exp(j*Vac_Init(2)*pi/180);
      | u2=Vdc_Init*exp(j*90*pi/180);
      | u=u1+u2;
      | u0=imag(u); % input at  t=0;
      | I=eye(size(Ac));
      | sI1=I*j*(2*pi*Vac_Init(3));
      | sI2=I*j*0;
      | x=inv(sI1-Ac)*Bc*u1 + inv(sI2-Ac)*Bc*u2;
      | x0c=imag(x);
      | else
      | x0c=0;
      | end
      | %
      | if PlotResponse==1 % Plot frequency and step response
      | t=[0:Tc/1000:7*Tc];
      | f=param1(1):param1(3):param1(2);
      | w=2*pi*f;
      | switch FilterType
      | 	case 1, % Lowpass
      | 		Ystep=1 - exp(-t/Tc);
      | 		RepFreq=1./(1+Tc*j.*w);
      | 	case 2,   % Highpass
      | 		Ystep=exp(-t/Tc);
      | 		RepFreq=1./(1 + (1./(Tc*j.*w)));
      | end
      | %
      | Mag=abs(RepFreq);
      | Pha=angle(RepFreq)*180/pi;
      | %
      | figure(1)
      | subplot(2,1,1)
      | plot(f,Mag)
      | grid
      | title('Bode Diagram')
      | ylabel('Magnitude')
      | subplot(2,1,2)
      | plot(f,Pha)
      | ylabel('Phase (deg)')
      | xlabel('Frequency (Hz)')
      | grid
      | figure(2)
      | plot(t,Ystep)
      | grid
      | ylabel('Amplitude')
      | xlabel('Time (s)')
      | title('Step Response')
      | end
      | power_initmask();
      mask Help: This block is part of a subset of blocks in the Extras library that does not have documentation associated with it, other than the block mask description.
      mask TypeOptions FilterType: Lowpass | Highpass
      mask Callback Initialize: %parametres=get_param(gcb,'MaskValues');p3=parametres{3};p6=parametres{6};if strcmp(p3,'on');param4='on';param5='on';else;param4='off';param5='off';end;if strcmp(p6,'on');param7='on';else;param7='off';end;visible={'on','on','on',param4,param5,'on',param7};set_param(gcb,'MaskVisibilities',visible)
      mask Callback PlotResponse: %parametres=get_param(gcb,'MaskValues');p3=parametres{3};p6=parametres{6};if strcmp(p3,'on');param4='on';param5='on';else;param4='off';param5='off';end;if strcmp(p6,'on');param7='on';else;param7='off';end;visible={'on','on','on',param4,param5,'on',param7};set_param(gcb,'MaskVisibilities',visible)
      mask Display: plot(X,Y);
  Constant11 : Constant  Value=2
  Integrator : Integrator  LimitOutput=on  UpperSaturationLimit=UpperLimit  LowerSaturationLimit=LowerLimit  AbsoluteTolerance=1e-4
  Kp4 : Gain  Gain=Kp_Vac_SH  SaturateOnIntegerOverflow=on  OutDataTypeStr=Inherit: Same as input  ParamDataTypeStr=Inherit: Same as input
  Kp5 : Gain  Gain=Ki_Vac_SH  SaturateOnIntegerOverflow=on  OutDataTypeStr=Inherit: Same as input  ParamDataTypeStr=Inherit: Same as input
  Kp6 : Gain  Gain=Droop  SaturateOnIntegerOverflow=on  OutDataTypeStr=Inherit: Same as input  ParamDataTypeStr=Inherit: Same as input
  Memory2 : Memory
  Rate Limiter : RateLimiter  RisingSlewLimit=MaxRateChangeVref_SH  FallingSlewLimit=-MaxRateChangeVref_SH
  Relational Operator : RelationalOperator  Operator===  RndMeth=Nearest
  Saturation1 : Saturate  UpperLimit=UpperLimit  LowerLimit=LowerLimit
  Scope : Scope
  Sum1 : Sum  Inputs=|-+  InputSameDT=on  SaturateOnIntegerOverflow=on  OutDataTypeStr=Inherit: Same as first input
  Sum6 : Sum  InputSameDT=on  SaturateOnIntegerOverflow=on  OutDataTypeStr=Inherit: Same as first input
  Sum7 : Sum  Inputs=|+-  InputSameDT=on  SaturateOnIntegerOverflow=on  OutDataTypeStr=Inherit: Same as first input
  Switch : Switch  Threshold=0.5  SaturateOnIntegerOverflow=on
  Iqref : Outport  InitialOutput=0  VectorParamsAs1DForOutWhenUnconnected=off
  Vref* : Outport  Port=2  VectorParamsAs1DForOutWhenUnconnected=off
  wires:
  Integrator/1 -> Sum6/2
  Kp4/1 -> Sum6/1
  Sum6/1 -> Saturation1/1  "Iq_Ref"
  Kp5/1 -> Integrator/1
  Sum7/1 -> Kp5/1, Kp4/1
  Vm/1 -> Sum1/1, Switch/3
  Sum1/1 -> Sum7/1  "Err"
  Memory2/1 -> Switch/2
  Relational Operator/1 -> Memory2/1
  Constant11/1 -> Relational Operator/2
  OpMode/1 -> Relational Operator/1
  Switch/1 -> Rate Limiter/1
  Vref/1 -> Switch/1
  Rate Limiter/1 -> Vref*/1, Sum1/2
  Kp6/1 -> 1st-Order Filter/1(In)
  1st-Order Filter/1(Out) -> Sum7/2
  Saturation1/1 -> Scope/1, Iqref/1, Kp6/1

== system power_kundur_statcom01/100 MVA STATCOM1/statcom_control/Current Regulator ==
  note: Current Regulator
  note: Id positive(+) flowing into converter ==> Converter absorbing real power = P positive(+)
  note: Sign convention:
  note: Iq negative(-) flowing into converter (inductive current) ==> Converter absorbing reactive power = Q positive(+)
  Idq_ref : Inport
  Idq : Inport  Port=2
  Vdq : Inport  Port=3
  Demux : Demux  Outputs=2
      settings: DisplayOption=none
  Demux1 : Demux  Outputs=2
      settings: DisplayOption=none
  Demux2 : Demux  Outputs=2
      settings: DisplayOption=none
  Lchoke1 : Constant  Value=Kf_I
  Mux : Mux  Inputs=2
  PI : Subsystem
  PI1 : Subsystem
  Product : Product  InputSameDT=on  SaturateOnIntegerOverflow=on  OutDataTypeStr=Inherit: Same as first input
  Product1 : Product  InputSameDT=on  SaturateOnIntegerOverflow=on  OutDataTypeStr=Inherit: Same as first input
  Sum1 : Sum  Inputs=|+-  InputSameDT=on  SaturateOnIntegerOverflow=on  OutDataTypeStr=Inherit: Same as first input
  Sum2 : Sum  Inputs=-+|  InputSameDT=on  SaturateOnIntegerOverflow=on  OutDataTypeStr=Inherit: Same as first input
  Sum3 : Sum  Inputs=|++  InputSameDT=on  SaturateOnIntegerOverflow=on  OutDataTypeStr=Inherit: Same as first input
  Sum4 : Sum  Inputs=|+-  InputSameDT=on  SaturateOnIntegerOverflow=on  OutDataTypeStr=Inherit: Same as first input
  Sum5 : Sum  Inputs=|+-  InputSameDT=on  SaturateOnIntegerOverflow=on  OutDataTypeStr=Inherit: Same as first input
  Sum6 : Sum  Inputs=|-+  InputSameDT=on  SaturateOnIntegerOverflow=on  OutDataTypeStr=Inherit: Same as first input
  Vdq* : Outport  VectorParamsAs1DForOutWhenUnconnected=off
  wires:
  Sum4/1 -> PI/1(In1)
  PI/1(Out1) -> Sum1/2  "vd'"
  Product/1 -> Sum3/2
  PI1/1(Out1) -> Sum6/1  "vq'"
  Product1/1 -> Sum5/2
  Mux/1 -> Vdq*/1
  Sum1/1 -> Mux/1
  Sum6/1 -> Mux/2
  Idq/1 -> Demux/1
  Demux/1 -> Sum4/2, Product1/1  "Id"
  Demux/2 -> Sum2/1, Product/2  "Iq"
  Sum2/1 -> PI1/1(In1)
  Demux1/1 -> Sum4/1  "Id_ref"
  Idq_ref/1 -> Demux1/1
  Demux1/2 -> Sum2/2  "Iq_ref"
  Demux2/2 -> Sum5/1  "Vq"
  Demux2/1 -> Sum3/1  "Vd"
  Sum3/1 -> Sum1/1
  Sum5/1 -> Sum6/2
  Lchoke1/1 -> Product/1, Product1/2
  Vdq/1 -> Demux2/1

== system power_kundur_statcom01/100 MVA STATCOM1/statcom_control/Current Limiter1 ==
  note: up to 3% overload
      | on current magnitude
      | is allowed
  Iqref : Inport
  Id_avg : Inport  Port=2
  " 200 pu/s" : RateLimiter  RisingSlewLimit=200  FallingSlewLimit=-200
  (pu) : Constant  Value=1.03
  Math Function1 : Math  Operator=square  SignedPower=on  SaturateOnIntegerOverflow=on
  Math Function2 : Math  Operator=square  SignedPower=on  SaturateOnIntegerOverflow=on
  Math Function3 : Math  Operator=sqrt  SignedPower=on  SaturateOnIntegerOverflow=on
  Math Function4 : Math  Operator=square  SignedPower=on  SaturateOnIntegerOverflow=on
  MinMax : MinMax  Inputs=2  InputSameDT=on  SaturateOnIntegerOverflow=on  ZeroCross=off
  Product1 : Product  SaturateOnIntegerOverflow=on  OutDataTypeStr=Inherit: Same as first input
  Saturation : Saturate  UpperLimit=1e6  LowerLimit=0
  Sign : Signum
  Sum : Sum  Inputs=+-  SaturateOnIntegerOverflow=on
  Iqref* : Outport  VectorParamsAs1DForOutWhenUnconnected=off
  wires:
  " 200 pu/s"/1 -> Iqref*/1
  Iqref/1 -> Sign/1, Math Function4/1
  Saturation/1 -> Math Function3/1
  Math Function2/1 -> Sum/1
  (pu)/1 -> Math Function2/1
  Math Function1/1 -> Sum/2
  Sum/1 -> MinMax/1
  MinMax/1 -> Saturation/1
  Math Function4/1 -> MinMax/2
  Sign/1 -> Product1/2
  Math Function3/1 -> Product1/1
  Product1/1 -> " 200 pu/s"/1
  Id_avg/1 -> Math Function1/1

== system power_kundur_statcom01/100 MVA STATCOM1/statcom_control/DC Voltage Regulator ==
  Vdc : Inport
  Vdc_Ref : Inport  Port=2
  -1<Id<+1 : Saturate  UpperLimit=1  LowerLimit=-1
  Integrator : Integrator  LimitOutput=on  UpperSaturationLimit=1  LowerSaturationLimit=-1  AbsoluteTolerance=1e-4
  Kp4 : Gain  Gain=Kp  SaturateOnIntegerOverflow=on  OutDataTypeStr=Inherit: Same as input  ParamDataTypeStr=Inherit: Same as input
  Kp5 : Gain  Gain=Ki  SaturateOnIntegerOverflow=on  OutDataTypeStr=Inherit: Same as input  ParamDataTypeStr=Inherit: Same as input
  Sum : Sum  Inputs=|+-  InputSameDT=on  SaturateOnIntegerOverflow=on  OutDataTypeStr=Inherit: Same as first input
  Sum6 : Sum  InputSameDT=on  SaturateOnIntegerOverflow=on  OutDataTypeStr=Inherit: Same as first input
  Id_Ref : Outport  InitialOutput=0  VectorParamsAs1DForOutWhenUnconnected=off
  wires:
  -1<Id<+1/1 -> Id_Ref/1
  Sum6/1 -> -1<Id<+1/1
  Sum/1 -> Kp5/1, Kp4/1
  Integrator/1 -> Sum6/2
  Kp4/1 -> Sum6/1
  Kp5/1 -> Integrator/1
  Vdc_Ref/1 -> Sum/1
  Vdc/1 -> Sum/2

== system power_kundur_statcom01/100 MVA STATCOM1/statcom_control/Iqref Selection ==
  note: 2=Auto
  Vm : Inport  PortDimensions=1
  IqrefAuto : Inport  Port=2
  OpMode : Inport  Port=3
  Qref : Inport  Port=4  PortDimensions=1
  -1<Iq<+1 : Saturate  UpperLimit=1  LowerLimit=-1
  Avoid division by 0 : Saturate  UpperLimit=1e6  LowerLimit=1e-5
  Constant11 : Constant  Value=2
  Deg->Rad1 : Gain  Gain=-1  SaturateOnIntegerOverflow=on  OutDataTypeStr=Inherit: Same as input  ParamDataTypeStr=Inherit: Same as input
  Memory1 : Memory
  Product : Product  Inputs=*/  InputSameDT=on  SaturateOnIntegerOverflow=on  OutDataTypeStr=Inherit: Same as first input
  Rate Limiter1 : RateLimiter  RisingSlewLimit=MaxRateChangeQref_SH  FallingSlewLimit=-MaxRateChangeQref_SH
  Relational Operator1 : RelationalOperator  Operator===  RndMeth=Nearest  InputSameDT=on
  Switch : Switch  Threshold=0.5  SaturateOnIntegerOverflow=on  InputSameDT=on
  Iqref* : Outport  VectorParamsAs1DForOutWhenUnconnected=off
  wires:
  -1<Iq<+1/1 -> Switch/3
  Vm/1 -> Avoid division by 0/1
  Deg->Rad1/1 -> -1<Iq<+1/1
  Product/1 -> Deg->Rad1/1
  Avoid division by 0/1 -> Product/2
  Constant11/1 -> Relational Operator1/2
  OpMode/1 -> Relational Operator1/1
  Switch/1 -> Iqref*/1
  IqrefAuto/1 -> Switch/1
  Relational Operator1/1 -> Switch/2
  Qref/1 -> Memory1/1
  Memory1/1 -> Rate Limiter1/1
  Rate Limiter1/1 -> Product/1

== system power_kundur_statcom01/100 MVA STATCOM1/statcom_control/Vd_Vq--> m,Phi ==
  note: to limit the modulation
      | index (m) to 1
  note: For a three-level inverter:
      | V L-L rms = m * sqrt(3)/(2*sqrt(2)) * Vdc
  note: Convert Vd_Vq (pu/Vnom) --> modulation Index (m, phi)
      | and limit the value of m to 1
  note: The "K_Vdq2m" ratio is used to convert Vd_Vq values (based in pu/Vnom)
      | to m and phi values that will produce the desired Vd_Vq. This ratio is
      | computed in the STATCOM top level mask.
  VdVq : Inport
  0<m<1 : Saturate  UpperLimit=1  LowerLimit=0
  Cartesian to Polar : simulink_extras/Transformations/Cartesian to Polar
      settings: SourceProductName=Simulink Extras
  Demux : Demux  Outputs=2
      settings: DisplayOption=none
  Kp5 : Gain  Gain=K_Vdq2m_SH  SaturateOnIntegerOverflow=on  OutDataTypeStr=Inherit: Same as input  ParamDataTypeStr=Inherit: Same as input
  m : Outport  VectorParamsAs1DForOutWhenUnconnected=off
  phi : Outport  Port=2  VectorParamsAs1DForOutWhenUnconnected=off
  wires:
  VdVq/1 -> Kp5/1
  Cartesian to Polar/1 -> 0<m<1/1
  Demux/1 -> Cartesian to Polar/1
  Demux/2 -> Cartesian to Polar/2
  Kp5/1 -> Demux/1
  0<m<1/1 -> m/1
  Cartesian to Polar/2 -> phi/1

== system power_kundur_statcom01/100 MVA STATCOM1/Measurement System/STATCOM Measurement System/Mean Value (linear) ==
  note: 1 - exp(-T*s)
  note: __________
  note: T * s
  note: Implements the following expression
      | (using the Pade fonction):
  note: Out =
  note: * In
  note: __________________________________________________________________
  note: |
      | |
      | |
      | |
      | |
      | |
      | |
  In : Inport
  Gain1 : Gain  Gain=Freq  SaturateOnIntegerOverflow=on  OutDataTypeStr=Inherit: Same as input  ParamDataTypeStr=Inherit: Same as input
  Integrator : Integrator  InitialCondition=Vinit
  Pade approximation of 1 cycle delay : StateSpace  A=Ac  B=Bc  C=Cc  D=Dc  InitialCondition=x0c
  Sum : Sum  Inputs=|+-  SaturateOnIntegerOverflow=on
  Mean : Outport  VectorParamsAs1DForOutWhenUnconnected=off
  wires:
  Integrator/1 -> Mean/1  "Mean value"
  Gain1/1 -> Integrator/1
  In/1 -> Sum/1, Pade approximation of 1 cycle delay/1
  Pade approximation of 1 cycle delay/1 -> Sum/2
  Sum/1 -> Gain1/1

== system power_kundur_statcom01/100 MVA STATCOM1/Measurement System/STATCOM Measurement System/Mean Value (linear)1 ==
  note: 1 - exp(-T*s)
  note: __________
  note: T * s
  note: Implements the following expression
      | (using the Pade fonction):
  note: Out =
  note: * In
  note: __________________________________________________________________
  note: |
      | |
      | |
      | |
      | |
      | |
      | |
  In : Inport
  Gain1 : Gain  Gain=Freq  SaturateOnIntegerOverflow=on  OutDataTypeStr=Inherit: Same as input  ParamDataTypeStr=Inherit: Same as input
  Integrator : Integrator  InitialCondition=Vinit
  Pade approximation of 1 cycle delay : StateSpace  A=Ac  B=Bc  C=Cc  D=Dc  InitialCondition=x0c
  Sum : Sum  Inputs=|+-  SaturateOnIntegerOverflow=on
  Mean : Outport  VectorParamsAs1DForOutWhenUnconnected=off
  wires:
  Integrator/1 -> Mean/1  "Mean value"
  Gain1/1 -> Integrator/1
  In/1 -> Sum/1, Pade approximation of 1 cycle delay/1
  Pade approximation of 1 cycle delay/1 -> Sum/2
  Sum/1 -> Gain1/1

== system power_kundur_statcom01/100 MVA STATCOM1/Measurement System/STATCOM Measurement System/Mean Value (linear)2 ==
  note: 1 - exp(-T*s)
  note: __________
  note: T * s
  note: Implements the following expression
      | (using the Pade fonction):
  note: Out =
  note: * In
  note: __________________________________________________________________
  note: |
      | |
      | |
      | |
      | |
      | |
      | |
  In : Inport
  Gain1 : Gain  Gain=Freq  SaturateOnIntegerOverflow=on  OutDataTypeStr=Inherit: Same as input  ParamDataTypeStr=Inherit: Same as input
  Integrator : Integrator  InitialCondition=Vinit
  Pade approximation of 1 cycle delay : StateSpace  A=Ac  B=Bc  C=Cc  D=Dc  InitialCondition=x0c
  Sum : Sum  Inputs=|+-  SaturateOnIntegerOverflow=on
  Mean : Outport  VectorParamsAs1DForOutWhenUnconnected=off
  wires:
  Integrator/1 -> Mean/1  "Mean value"
  Gain1/1 -> Integrator/1
  In/1 -> Sum/1, Pade approximation of 1 cycle delay/1
  Pade approximation of 1 cycle delay/1 -> Sum/2
  Sum/1 -> Gain1/1

== system power_kundur_statcom01/100 MVA STATCOM1/Measurement System/STATCOM Measurement System/Q computation ==
  note: Q = Vq*Id - Vd*Iq
  Vdq : Inport
  Idq : Inport  Port=2
  Demux : Demux  Outputs=2
      settings: DisplayOption=none
  Product3 : Product  InputSameDT=on  SaturateOnIntegerOverflow=on  OutDataTypeStr=Inherit: Same as first input
  Selector : Selector  InputPortWidth=2  IndexOptions=Index vector (dialog)  Indices=[2 1]  OutputSizes=1
  Sum2 : Sum  Inputs=+-  InputSameDT=on  SaturateOnIntegerOverflow=on  OutDataTypeStr=Inherit: Same as first input
  Q : Outport  VectorParamsAs1DForOutWhenUnconnected=off
  wires:
  Demux/2 -> Sum2/2
  Demux/1 -> Sum2/1
  Product3/1 -> Demux/1
  Sum2/1 -> Q/1
  Idq/1 -> Product3/2
  Selector/1 -> Product3/1
  Vdq/1 -> Selector/1

== system power_kundur_statcom01/100 MVA STATCOM1/Power Components Modeling (Shunt & Series Converter)/Power Components modeling (Shunt Converter)/dq-axis model of 3-ph RL branch ==
  V1abc : Inport
  V2abc : Inport  Port=2
  R_RL : Inport  Port=3
  Positive-sequence d-q axis model of a 3-phase series R-L branch : Subsystem  mask(d-q axis model of a 3-phase series R-L branch){R=R_RL, L=L_RL, Fnom=Fnom}
      mask prompts: R "R (pu)"; L "L (pu)"; Fnom "Nominal frequency (Hz)"
      mask help:
      | This block implements a d-q axis model of a 3-phase R-L branch.
      | Inputs:
      | d-q axis voltages (V1 and V2) at each terminal of the R-L branch in pu.
      | Outputs:
      | d-q axis currents flowing (from V1 to V2) in the R-L branch in pu.
      mask init:
      | w=2*pi*Fnom;
  V-->pu : Gain  Gain=1/(Vnom*sqrt(2)/sqrt(3))  SaturateOnIntegerOverflow=on  OutDataTypeStr=Inherit: Same as input  ParamDataTypeStr=Inherit: Same as input
  "V-->pu " : Gain  Gain=1/(Vnom*sqrt(2)/sqrt(3))  SaturateOnIntegerOverflow=on  OutDataTypeStr=Inherit: Same as input  ParamDataTypeStr=Inherit: Same as input
  abc2dq : Subsystem
  abc2dq1 : Subsystem
  dq2ab : Subsystem
  pu-->A2 : Gain  Gain=Pnom*sqrt(2)/(sqrt(3)*Vnom)  SaturateOnIntegerOverflow=on  OutDataTypeStr=Inherit: Same as input  ParamDataTypeStr=Inherit: Same as input
  Ia_Ib : Outport  VectorParamsAs1DForOutWhenUnconnected=off
  wires:
  abc2dq1/1(Vdq_seq1) -> Positive-sequence d-q axis model of a 3-phase series R-L branch/2(Vdq2)
  abc2dq/1(Vdq_seq1) -> Positive-sequence d-q axis model of a 3-phase series R-L branch/1(Vdq1)
  V2abc/1 -> V-->pu/1
  pu-->A2/1 -> Ia_Ib/1
  V1abc/1 -> "V-->pu "/1
  "V-->pu "/1 -> abc2dq/1(Vabc cmplx)
  V-->pu/1 -> abc2dq1/1(Vabc cmplx)
  dq2ab/1(Ia_Ib complx) -> pu-->A2/1
  Positive-sequence d-q axis model of a 3-phase series R-L branch/1(idIq) -> dq2ab/1(Idq_seq1)  "Idq_seq1"
  R_RL/1 -> Positive-sequence d-q axis model of a 3-phase series R-L branch/3(R_RL)

== system power_kundur_statcom01/100 MVA STATCOM1/statcom_control/AC Voltage Regulator/1st-Order Filter ==
  In : Inport
  State-Space : StateSpace  A=Ac  B=Bc  C=Cc  D=Dc  InitialCondition=x0c
  Out : Outport  InitialOutput=0  VectorParamsAs1DForOutWhenUnconnected=off
  wires:
  State-Space/1 -> Out/1
  In/1 -> State-Space/1
